simulink model "test_DSSS_tranmission_receiver_chain_spectrum_analysis"  (R2016a)
settings: Solver=VariableStepAuto  StartTime=0.0  StopTime=20  RelTol=1e-3
libraries: commblkcod2 x2, commdigbbndpm3 x2, commsequence2 x2, commblkintrlv2 x2, commchan3 x1, commsink2 x1, commseqgen3 x1, commrandsrc3 x1, commutil2 x1
settings Model: Creator=malaika  LastModifiedBy=malaika

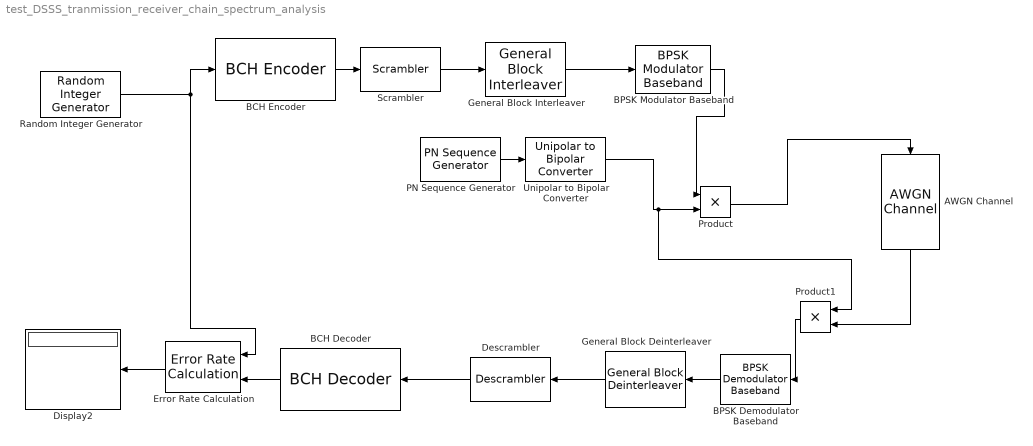
== system test_DSSS_tranmission_receiver_chain_spectrum_analysis ==
  AWGN Channel : commchan3/AWGN Channel  InputProcessing=Columns as channels (frame based)  seed=67  noiseMode="Signal to noise ratio  (Eb/No)"  EbNodB=100  EsNodB=10  SNRdB=10  bitsPerSym=1  Ps=1  Tsym=0.002  variance=1
  BCH Decoder : commblkcod2/BCH Decoder  n=15  k=5  specShortening=off  shortenedK=5  specGenPoly=off  genPoly='X^10 + X^8 + X^5 + X^4 + X^2 + X + 1'  specPrimPoly=on  prPoly='X^4 + X + 1'  specDisableGenCheck=off  specPuncture=off  punctVec=[ones(8,1); zeros(2,1)]  specErasurePort=off  showNumErr=off
  BCH Encoder : commblkcod2/BCH Encoder  n=15  k=5  specShortening=off  shortenedK=5  specGenPoly=off  genPoly='X^10 + X^8 + X^5 + X^4 + X^2 + X + 1'  specPrimPoly=on  prPoly='X^4 + X + 1'  specDisableGenCheck=off  specPuncture=off  punctVec=[ones(8,1); zeros(2,1)]
  BPSK Demodulator Baseband : commdigbbndpm3/BPSK Demodulator Baseband  DecType=Hard decision  VarSource=Dialog  Variance=1  Ph=0  outDtype=double  derotateFactorWordLen=16  derotateFactorDataTypeStr=Inherit: Same word length as input  derotateFactorLastDataTypeStr=Inherit: Same word length as input
  BPSK Modulator Baseband : commdigbbndpm3/BPSK Modulator Baseband  Ph=0  outDtype=double  outWordLen=16  outUDDataType=sfix(16)  outFracLenMode=Best precision  outFracLen=15  outDataTypeStr=double  outLastDataTypeStr=double
  Descrambler : commsequence2/Descrambler  M=2  poly='1 + z^-1 + z^-2 + z^-4'  iniStaSource=Dialog Parameter  ini_sta=[0 1 0 1]  resetViaPort=off
  Display2 : Display
  Error Rate Calculation : commsink2/Error Rate Calculation  N=0  st_delay=0  cp_mode=Entire frame  subframe=[]  PMode=Port  WsName=ErrorVec  RsMode2=off  stop=off  numErr=100  maxBits=1e6
  General Block Deinterleaver : commblkintrlv2/General Block Deinterleaver  permutationVectorSource=Dialog  elements=[15:-1:1].'
  General Block Interleaver : commblkintrlv2/General Block Interleaver  permutationVectorSource=Dialog  elements=[15:-1:1].'
  PN Sequence Generator : commseqgen3/PN Sequence Generator  poly='z^6 + z + 1'  ini_sta=[1 0 0 0 0 1]  outBitMaskSource=Dialog parameter  shift=0  outVarSiz=off  maxOutSizeMode=Dialog parameter  maxOutSize=[10 1]  Ts=0.002  sampPerFrame=15  reset=off  bitPackedOutputs=off  outDataType=double  numPackedBits=8  bitPackDataSigned=off  bitPackedOutDType=double
  Product : Product
  Product1 : Product
  Random Integer Generator : commrandsrc3/Random Integer Generator  SetSize=2  SeedSource=Auto  Seed=0  SampleTime=0.002  SamplesPerFrame=5  OutputDataType=double  SimulateUsing=Interpreted execution
  Scrambler : commsequence2/Scrambler  M=2  poly='1 + z^-1 + z^-2 + z^-4'  iniStaSource=Dialog Parameter  ini_sta=[0 1 0 1]  resetViaPort=off
  Unipolar to Bipolar Converter : commutil2/Unipolar to Bipolar Converter  M=4  polarity=Positive  dataType=Inherit via internal rule
  wires:
  Random Integer Generator/1 -> BCH Encoder/1, Error Rate Calculation/1
  Error Rate Calculation/1 -> Display2/1
  BPSK Modulator Baseband/1 -> Product/1
  BPSK Demodulator Baseband/1 -> General Block Deinterleaver/1
  PN Sequence Generator/1 -> Unipolar to Bipolar Converter/1
  Unipolar to Bipolar Converter/1 -> Product1/1, Product/2
  Product/1 -> AWGN Channel/1
  AWGN Channel/1 -> Product1/2
  Product1/1 -> BPSK Demodulator Baseband/1
  BCH Encoder/1 -> Scrambler/1
  BCH Decoder/1 -> Error Rate Calculation/2
  Scrambler/1 -> General Block Interleaver/1
  Descrambler/1 -> BCH Decoder/1
  General Block Interleaver/1 -> BPSK Modulator Baseband/1
  General Block Deinterleaver/1 -> Descrambler/1
